simulink library "ROTH"  (R2016b)
settings: Solver=ode45  StartTime=0.0  StopTime=10.0  RelTol=1e-3  EnableMultiTasking=on
undefined symbols (not defined in the file): CAL_EAST, CAL_NORTH, CAL_SOUTH, CAL_WEST, CONST_EndOfLineEnableFlg, ENU_END, ENU_FORWARD, ENU_GTSP, ENU_LEFT_BUSY_RIGHT_BUSY, ENU_LEFT_BUSY_RIGHT_CLEANED, ENU_LEFT_BUSY_RIGHT_EMPTY, ENU_LEFT_CLEANED_RIGHT_BUSY, ENU_LEFT_CLEANED_RIGHT_CLEANED, ENU_LEFT_CLEANED_RIGHT_EMPTY, ENU_LEFT_EMPTY_RIGHT_BUSY, ENU_LEFT_EMPTY_RIGHT_CLEANED, ENU_LEFT_EMPTY_RIGHT_EMPTY, ENU_MOVE_TURN_LEFT, ENU_MOVE_TURN_RIGHT, ENU_MOVE_U_TURN, ENU_MOVE_U_TURN_LEFT, ENU_MOVE_U_TURN_RIGHT, ENU_STOP, ENU_ZIGZAG
settings Model: Creator=oelkawok  LastModifiedBy=oelkawok
settings DataIOCC: LimitDataPoints=on
settings OptimizationCC: LifeSpan=inf
settings DebuggingCC: AllowSymbolicDim=off  SFUnexpectedBacktrackingDiag=warning  SFNoUnconditionalDefaultTransitionDiag=warning  SFExecutionAtInitializationDiag=none
settings GRTTargetCC: TargetLangStandard=C89/C90 (ANSI)  GeneratePreprocessorConditionals=Disable all
settings ConfigComp: CovMetricSettings=dw  CovHtmlReporting=on  CovSaveCumulativeToWorkspaceVar=on  CovSaveSingleToWorkspaceVar=on  CovExternalEMLEnable=off

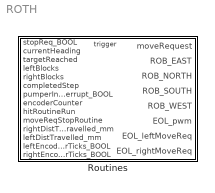
== system ROTH ==
  Routines : Subsystem

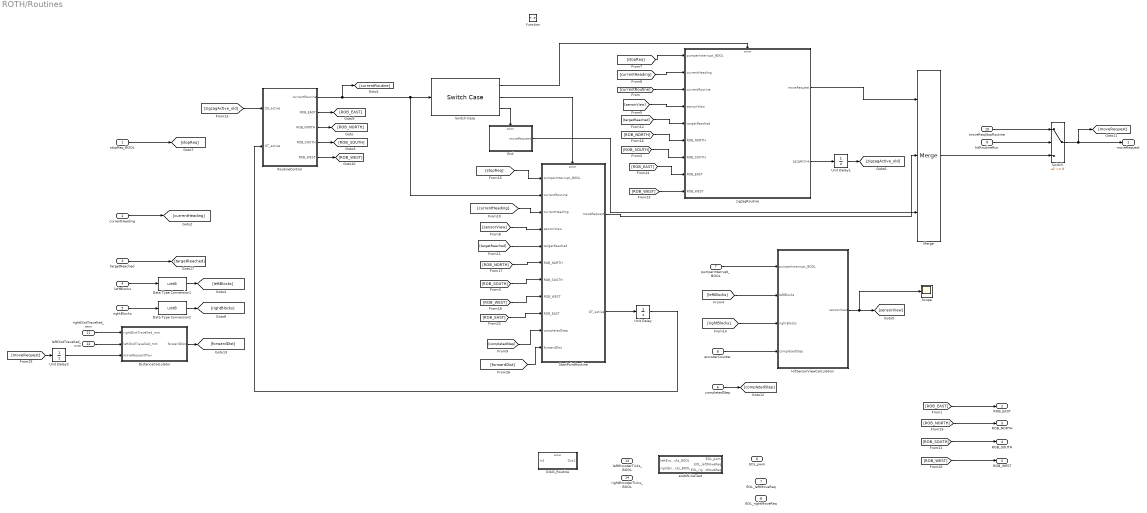
== system ROTH/Routines ==
  stopReq_BOOL : Inport
  currentHeading : Inport  Port=2
  targetReached : Inport  Port=3
  leftBlocks : Inport  Port=4
  rightBlocks : Inport  Port=5
  completedStep : Inport  Port=6
  pumperInterrupt_BOOL : Inport  Port=7
  encoderCounter : Inport  Port=8
  hitRoutineRun : Inport  Port=9
  moveReqStopRoutine : Inport  Port=10
  rightDistTravelled_mm : Inport  Port=11  PortDimensions=1
  leftDistTravelled_mm : Inport  Port=12  PortDimensions=1
  leftEncoderTicks_BOOL : Inport  Port=13  PortDimensions=1
  rightEncoderTicks_BOOL : Inport  Port=14  PortDimensions=1
  function : TriggerPort  TriggerType=function-call  VariantControl=Variant
  DIAG_Routine : Subsystem
  Data Type Conversion1 : DataTypeConversion  OutDataTypeStr=uint8
  Data Type Conversion2 : DataTypeConversion  OutDataTypeStr=uint8
  DistanceCalculator : Subsystem
  End : Subsystem  TreatAsAtomicUnit=on
  HitSensorViewCalculation : Subsystem
  Merge : Merge  Inputs=3  InitialOutput=5
      settings: AttributesFormatString=%<InitialOutput>
  RoutineControl : Subsystem
  Scope : Scope
  StartPointRoutine : Subsystem
  Switch : Switch  Criteria=u2 ~= 0
  Switch Case : SwitchCase  CaseConditions={ENU_ZIGZAG, ENU_GTSP, ENU_END}  ShowDefaultCase=off
      settings: AttributesFormatString=%<CaseConditions>
  Unit Delay : UnitDelay  InitialCondition=true  SampleTime=-1
      settings: AttributesFormatString=%<InitialCondition>
  Unit Delay1 : UnitDelay  InitialCondition=false  SampleTime=-1
      settings: AttributesFormatString=%<InitialCondition>
  Unit Delay2 : UnitDelay  SampleTime=-1
  endofLineTest : Subsystem
  zigzagRoutine : Subsystem
  moveRequest : Outport
  ROB_EAST : Outport  Port=2
  ROB_NORTH : Outport  Port=3
  ROB_SOUTH : Outport  Port=4
  ROB_WEST : Outport  Port=5
  EOL_pwm : Outport  Port=6
  EOL_leftMoveReq : Outport  Port=7
  EOL_rightMoveReq : Outport  Port=8
  wires:
  [forwardDist] -> StartPointRoutine/11(forwardDist)
  DistanceCalculator/1(forwardDist) -> [forwardDist]
  Unit Delay2/1 -> DistanceCalculator/3(moveRequestPrev)
  [moveRequest] -> Unit Delay2/1
  leftDistTravelled_mm/1 -> DistanceCalculator/2(leftDistTravelled_mm)
  rightDistTravelled_mm/1 -> DistanceCalculator/1(rightDistTravelled_mm)
  encoderCounter/1 -> HitSensorViewCalculation/4(completedStep)
  [ROB_WEST] -> zigzagRoutine/9(ROB_WEST)
  [ROB_EAST] -> zigzagRoutine/8(ROB_EAST)
  [completedStep] -> StartPointRoutine/10(completedStep)
  End/1(moveRequest) -> Merge/3
  Switch Case/3 -> End/Action
  [ROB_EAST] -> StartPointRoutine/9(ROB_EAST)
  [ROB_WEST] -> ROB_WEST/1
  [ROB_SOUTH] -> ROB_SOUTH/1
  [ROB_NORTH] -> ROB_NORTH/1
  [ROB_EAST] -> ROB_EAST/1
  [ROB_WEST] -> StartPointRoutine/8(ROB_WEST)
  [ROB_NORTH] -> StartPointRoutine/6(ROB_NORTH)
  [ROB_NORTH] -> zigzagRoutine/6(ROB_NORTH)
  [ROB_SOUTH] -> StartPointRoutine/7(ROB_SOUTH)
  [ROB_SOUTH] -> zigzagRoutine/7(ROB_SOUTH)
  RoutineControl/4(ROB_SOUTH) -> [ROB_SOUTH]
  RoutineControl/5(ROB_WEST) -> [ROB_WEST]
  RoutineControl/2(ROB_EAST) -> [ROB_EAST]
  RoutineControl/3(ROB_NORTH) -> [ROB_NORTH]
  stopReq_BOOL/1 -> [stopReq]
  [targetReached] -> zigzagRoutine/5(targetReached)
  [targetReached] -> StartPointRoutine/5(targetReached)
  targetReached/1 -> [targetReached]
  [currentHeading] -> StartPointRoutine/3(currentHeading)
  [sensorView] -> StartPointRoutine/4(sensorView)
  [stopReq] -> StartPointRoutine/1(pumperInterrupt_BOOL)
  zigzagRoutine/2(zgzgActive) -> Unit Delay1/1
  zigzagRoutine/1(moveRequest) -> Merge/1
  StartPointRoutine/1(moveRequest) -> Merge/2
  pumperInterrupt_BOOL/1 -> HitSensorViewCalculation/1(pumperInterrupt_BOOL)
  Switch Case/2 -> StartPointRoutine/Action
  Switch Case/1 -> zigzagRoutine/Action
  RoutineControl/1(currentRoutine) -> [currentRoutine], Switch Case/1, StartPointRoutine/2(currentRoutine)
  [currentHeading] -> zigzagRoutine/2(currentHeading)
  [stopReq] -> zigzagRoutine/1(pumperInterrupt_BOOL)
  [sensorView] -> zigzagRoutine/4(sensorView)
  HitSensorViewCalculation/1(sensorView) -> Scope/1, [sensorView]
  StartPointRoutine/2(GT_active) -> Unit Delay/1
  Unit Delay/1 -> RoutineControl/2(GT_active)
  currentHeading/1 -> [currentHeading]
  [currentRoutine] -> zigzagRoutine/3(currentRoutine)
  Unit Delay1/1 -> [zigzagActive_old]
  [zigzagActive_old] -> RoutineControl/1(ZG_active)
  leftBlocks/1 -> Data Type Conversion1/1
  rightBlocks/1 -> Data Type Conversion2/1
  Data Type Conversion1/1 -> [leftBlocks]
  Data Type Conversion2/1 -> [rightBlocks]
  [rightBlocks] -> HitSensorViewCalculation/3(rightBlocks)
  [leftBlocks] -> HitSensorViewCalculation/2(leftBlocks)
  completedStep/1 -> [completedStep]
  Switch/1 -> moveRequest/1, [moveRequest]
  moveReqStopRoutine/1 -> Switch/1
  hitRoutineRun/1 -> Switch/2
  Merge/1 -> Switch/3

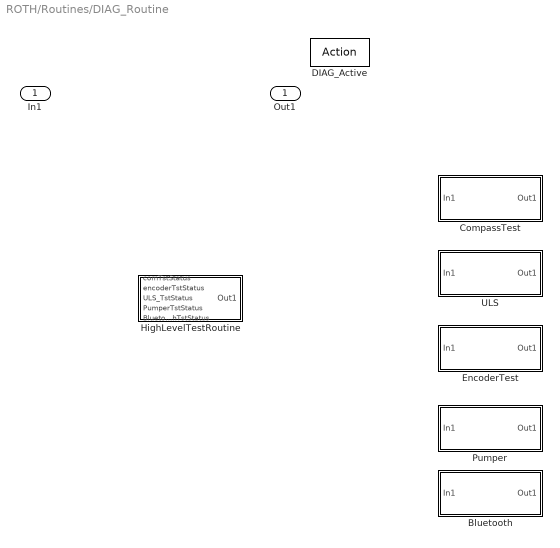
== system ROTH/Routines/DIAG_Routine ==
  In1 : Inport
  DIAG_Active : ActionPort
  Bluetooth : Subsystem
  CompassTest : Subsystem
  EncoderTest : Subsystem
  HighLevelTestRoutine : Subsystem
  Pumper : Subsystem
  ULS : Subsystem
  Out1 : Outport

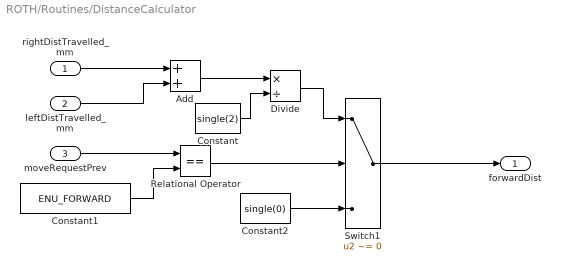
== system ROTH/Routines/DistanceCalculator ==
  rightDistTravelled_mm : Inport  PortDimensions=1
  leftDistTravelled_mm : Inport  Port=2  PortDimensions=1
  moveRequestPrev : Inport  Port=3  PortDimensions=1
  Add : Sum
  Constant : Constant  Value=single(2)
  Constant1 : Constant  Value=ENU_FORWARD
  Constant2 : Constant  Value=single(0)
  Divide : Product  Inputs=*/
  Relational Operator : RelationalOperator  Operator===  OutDataTypeStr=boolean  RndMeth=Simplest
  Switch1 : Switch  Criteria=u2 ~= 0
  forwardDist : Outport
  wires:
  Add/1 -> Divide/1
  moveRequestPrev/1 -> Relational Operator/1
  Constant2/1 -> Switch1/3
  leftDistTravelled_mm/1 -> Add/2
  rightDistTravelled_mm/1 -> Add/1
  Constant1/1 -> Relational Operator/2
  Switch1/1 -> forwardDist/1
  Divide/1 -> Switch1/1
  Relational Operator/1 -> Switch1/2
  Constant/1 -> Divide/2

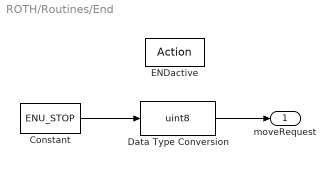
== system ROTH/Routines/End ==
  ENDactive : ActionPort
  Constant : Constant  Value=ENU_STOP
  Data Type Conversion : DataTypeConversion  OutDataTypeStr=uint8
  moveRequest : Outport
  wires:
  Data Type Conversion/1 -> moveRequest/1
  Constant/1 -> Data Type Conversion/1

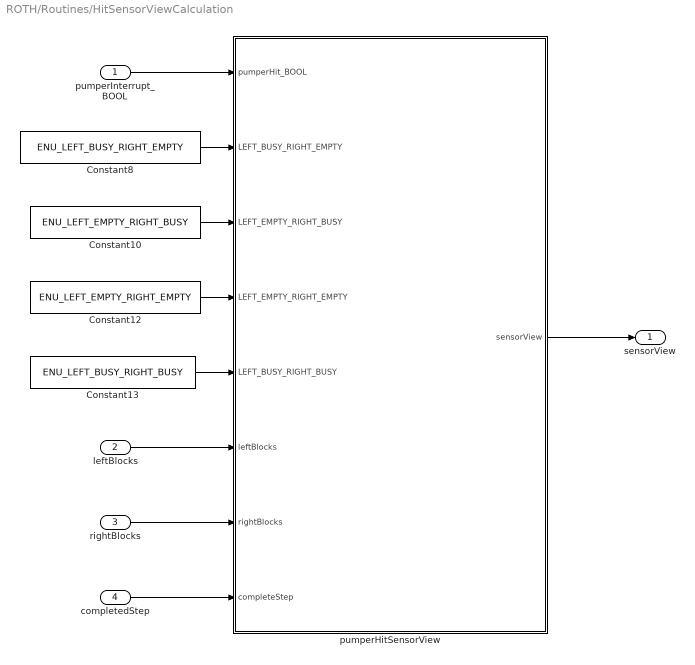
== system ROTH/Routines/HitSensorViewCalculation ==
  pumperInterrupt_BOOL : Inport
  leftBlocks : Inport  Port=2
  rightBlocks : Inport  Port=3
  completedStep : Inport  Port=4
  Constant10 : Constant  Value=ENU_LEFT_EMPTY_RIGHT_BUSY
  Constant12 : Constant  Value=ENU_LEFT_EMPTY_RIGHT_EMPTY
  Constant13 : Constant  Value=ENU_LEFT_BUSY_RIGHT_BUSY
  Constant8 : Constant  Value=ENU_LEFT_BUSY_RIGHT_EMPTY
  pumperHitSensorView : Stateflow chart  TreatAsAtomicUnit=on
  sensorView : Outport
  wires:
  pumperInterrupt_BOOL/1 -> pumperHitSensorView/1(pumperHit_BOOL)
  Constant8/1 -> pumperHitSensorView/2(LEFT_BUSY_RIGHT_EMPTY)
  Constant10/1 -> pumperHitSensorView/3(LEFT_EMPTY_RIGHT_BUSY)
  Constant12/1 -> pumperHitSensorView/4(LEFT_EMPTY_RIGHT_EMPTY)
  Constant13/1 -> pumperHitSensorView/5(LEFT_BUSY_RIGHT_BUSY)
  pumperHitSensorView/1(sensorView) -> sensorView/1
  leftBlocks/1 -> pumperHitSensorView/6(leftBlocks)
  rightBlocks/1 -> pumperHitSensorView/7(rightBlocks)
  completedStep/1 -> pumperHitSensorView/8(completeStep)

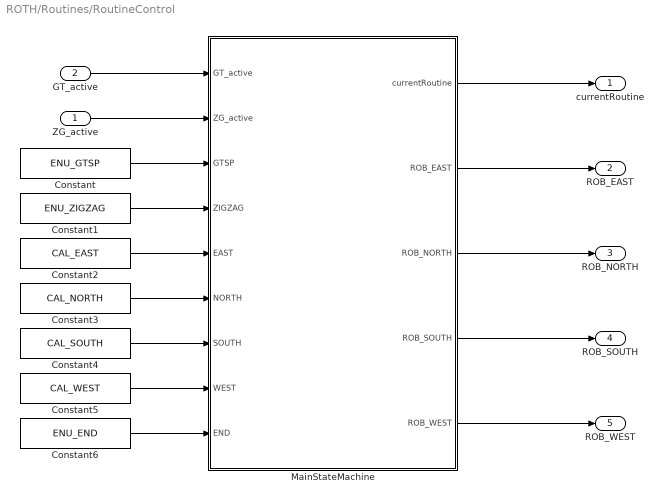
== system ROTH/Routines/RoutineControl ==
  ZG_active : Inport
  GT_active : Inport  Port=2
  Constant : Constant  Value=ENU_GTSP
  Constant1 : Constant  Value=ENU_ZIGZAG
  Constant2 : Constant  Value=CAL_EAST
  Constant3 : Constant  Value=CAL_NORTH
  Constant4 : Constant  Value=CAL_SOUTH
  Constant5 : Constant  Value=CAL_WEST
  Constant6 : Constant  Value=ENU_END
  MainStateMachine : Stateflow chart  TreatAsAtomicUnit=on
  currentRoutine : Outport
  ROB_EAST : Outport  Port=2
  ROB_NORTH : Outport  Port=3
  ROB_SOUTH : Outport  Port=4
  ROB_WEST : Outport  Port=5
  wires:
  Constant6/1 -> MainStateMachine/9(END)
  MainStateMachine/5(ROB_WEST) -> ROB_WEST/1
  MainStateMachine/4(ROB_SOUTH) -> ROB_SOUTH/1
  MainStateMachine/3(ROB_NORTH) -> ROB_NORTH/1
  MainStateMachine/2(ROB_EAST) -> ROB_EAST/1
  Constant4/1 -> MainStateMachine/7(SOUTH)
  Constant3/1 -> MainStateMachine/6(NORTH)
  Constant5/1 -> MainStateMachine/8(WEST)
  Constant2/1 -> MainStateMachine/5(EAST)
  ZG_active/1 -> MainStateMachine/2(ZG_active)
  GT_active/1 -> MainStateMachine/1(GT_active)
  MainStateMachine/1(currentRoutine) -> currentRoutine/1
  Constant/1 -> MainStateMachine/3(GTSP)
  Constant1/1 -> MainStateMachine/4(ZIGZAG)

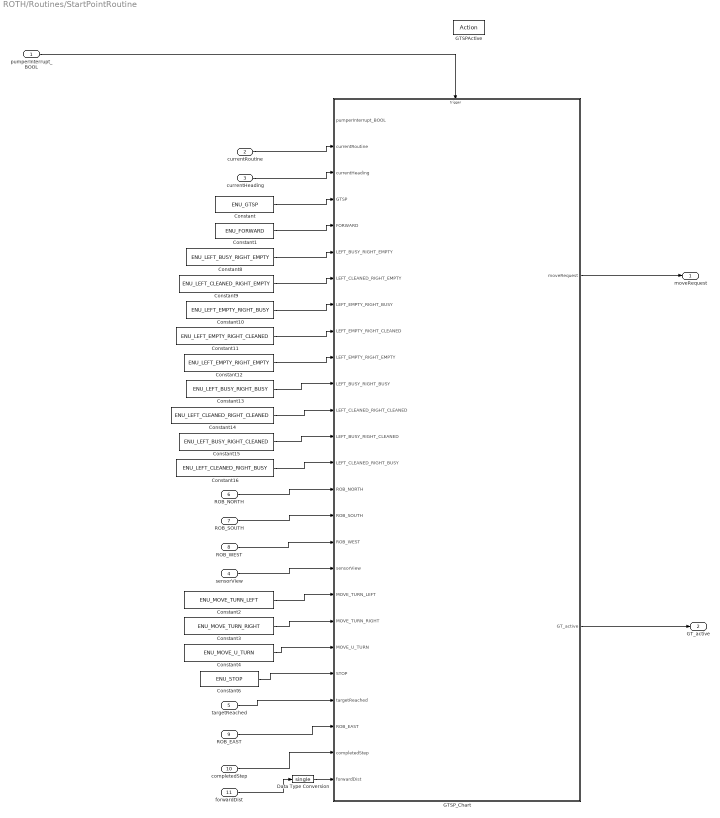
== system ROTH/Routines/StartPointRoutine ==
  pumperInterrupt_BOOL : Inport
  currentRoutine : Inport  Port=2
  currentHeading : Inport  Port=3
  sensorView : Inport  Port=4
  targetReached : Inport  Port=5
  ROB_NORTH : Inport  Port=6
  ROB_SOUTH : Inport  Port=7
  ROB_WEST : Inport  Port=8
  ROB_EAST : Inport  Port=9
  completedStep : Inport  Port=10
  forwardDist : Inport  Port=11
  GTSPActive : ActionPort
  Constant : Constant  Value=ENU_GTSP
  Constant1 : Constant  Value=ENU_FORWARD
  Constant10 : Constant  Value=ENU_LEFT_EMPTY_RIGHT_BUSY
  Constant11 : Constant  Value=ENU_LEFT_EMPTY_RIGHT_CLEANED
  Constant12 : Constant  Value=ENU_LEFT_EMPTY_RIGHT_EMPTY
  Constant13 : Constant  Value=ENU_LEFT_BUSY_RIGHT_BUSY
  Constant14 : Constant  Value=ENU_LEFT_CLEANED_RIGHT_CLEANED
  Constant15 : Constant  Value=ENU_LEFT_BUSY_RIGHT_CLEANED
  Constant16 : Constant  Value=ENU_LEFT_CLEANED_RIGHT_BUSY
  Constant2 : Constant  Value=ENU_MOVE_TURN_LEFT
  Constant3 : Constant  Value=ENU_MOVE_TURN_RIGHT
  Constant4 : Constant  Value=ENU_MOVE_U_TURN
  Constant6 : Constant  Value=ENU_STOP
  Constant8 : Constant  Value=ENU_LEFT_BUSY_RIGHT_EMPTY
  Constant9 : Constant  Value=ENU_LEFT_CLEANED_RIGHT_EMPTY
  Data Type Conversion : DataTypeConversion  OutDataTypeStr=single
  GTSP_Chart : Stateflow chart  TreatAsAtomicUnit=on
  moveRequest : Outport
  GT_active : Outport  Port=2
  wires:
  Data Type Conversion/1 -> GTSP_Chart/26(forwardDist)
  forwardDist/1 -> Data Type Conversion/1
  completedStep/1 -> GTSP_Chart/25(completedStep)
  pumperInterrupt_BOOL/1 -> GTSP_Chart/Trigger
  GTSP_Chart/1(moveRequest) -> moveRequest/1
  ROB_EAST/1 -> GTSP_Chart/24(ROB_EAST)
  targetReached/1 -> GTSP_Chart/23(targetReached)
  currentHeading/1 -> GTSP_Chart/3(currentHeading)
  currentRoutine/1 -> GTSP_Chart/2(currentRoutine)
  Constant/1 -> GTSP_Chart/4(GTSP)
  Constant1/1 -> GTSP_Chart/5(FORWARD)
  Constant8/1 -> GTSP_Chart/6(LEFT_BUSY_RIGHT_EMPTY)
  Constant9/1 -> GTSP_Chart/7(LEFT_CLEANED_RIGHT_EMPTY)
  Constant10/1 -> GTSP_Chart/8(LEFT_EMPTY_RIGHT_BUSY)
  Constant11/1 -> GTSP_Chart/9(LEFT_EMPTY_RIGHT_CLEANED)
  Constant12/1 -> GTSP_Chart/10(LEFT_EMPTY_RIGHT_EMPTY)
  Constant13/1 -> GTSP_Chart/11(LEFT_BUSY_RIGHT_BUSY)
  Constant14/1 -> GTSP_Chart/12(LEFT_CLEANED_RIGHT_CLEANED)
  Constant15/1 -> GTSP_Chart/13(LEFT_BUSY_RIGHT_CLEANED)
  Constant16/1 -> GTSP_Chart/14(LEFT_CLEANED_RIGHT_BUSY)
  ROB_WEST/1 -> GTSP_Chart/17(ROB_WEST)
  ROB_SOUTH/1 -> GTSP_Chart/16(ROB_SOUTH)
  ROB_NORTH/1 -> GTSP_Chart/15(ROB_NORTH)
  sensorView/1 -> GTSP_Chart/18(sensorView)
  Constant4/1 -> GTSP_Chart/21(MOVE_U_TURN)
  Constant3/1 -> GTSP_Chart/20(MOVE_TURN_RIGHT)
  Constant2/1 -> GTSP_Chart/19(MOVE_TURN_LEFT)
  GTSP_Chart/2(GT_active) -> GT_active/1
  Constant6/1 -> GTSP_Chart/22(STOP)

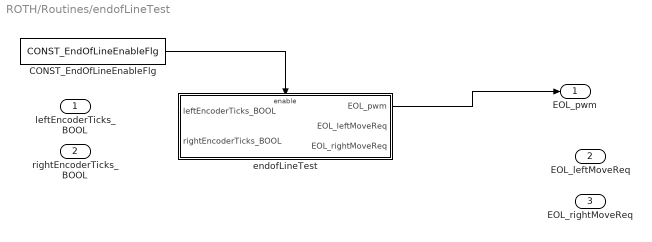
== system ROTH/Routines/endofLineTest ==
  leftEncoderTicks_BOOL : Inport  PortDimensions=1
  rightEncoderTicks_BOOL : Inport  Port=2  PortDimensions=1
  CONST_EndOfLineEnableFlg : Constant  Value=CONST_EndOfLineEnableFlg
  endofLineTest : Subsystem
  EOL_pwm : Outport
  EOL_leftMoveReq : Outport  Port=2
  EOL_rightMoveReq : Outport  Port=3
  wires:
  endofLineTest/1(EOL_pwm) -> EOL_pwm/1
  CONST_EndOfLineEnableFlg/1 -> endofLineTest/Enable

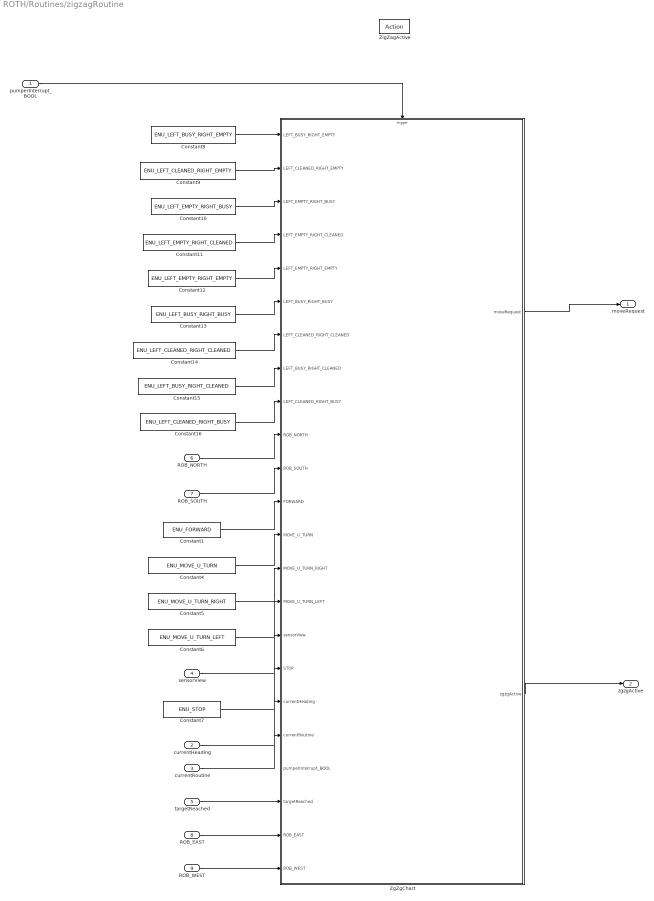
== system ROTH/Routines/zigzagRoutine ==
  pumperInterrupt_BOOL : Inport
  currentHeading : Inport  Port=2
  currentRoutine : Inport  Port=3
  sensorView : Inport  Port=4
  targetReached : Inport  Port=5
  ROB_NORTH : Inport  Port=6
  ROB_SOUTH : Inport  Port=7
  ROB_EAST : Inport  Port=8
  ROB_WEST : Inport  Port=9
  ZigZagActive : ActionPort
  Constant1 : Constant  Value=ENU_FORWARD
  Constant10 : Constant  Value=ENU_LEFT_EMPTY_RIGHT_BUSY
  Constant11 : Constant  Value=ENU_LEFT_EMPTY_RIGHT_CLEANED
  Constant12 : Constant  Value=ENU_LEFT_EMPTY_RIGHT_EMPTY
  Constant13 : Constant  Value=ENU_LEFT_BUSY_RIGHT_BUSY
  Constant14 : Constant  Value=ENU_LEFT_CLEANED_RIGHT_CLEANED
  Constant15 : Constant  Value=ENU_LEFT_BUSY_RIGHT_CLEANED
  Constant16 : Constant  Value=ENU_LEFT_CLEANED_RIGHT_BUSY
  Constant4 : Constant  Value=ENU_MOVE_U_TURN
  Constant5 : Constant  Value=ENU_MOVE_U_TURN_RIGHT
  Constant6 : Constant  Value=ENU_MOVE_U_TURN_LEFT
  Constant7 : Constant  Value=ENU_STOP
  Constant8 : Constant  Value=ENU_LEFT_BUSY_RIGHT_EMPTY
  Constant9 : Constant  Value=ENU_LEFT_CLEANED_RIGHT_EMPTY
  ZgZgChart : Stateflow chart  TreatAsAtomicUnit=on
  moveRequest : Outport
  zgzgActive : Outport  Port=2  InitialOutput=true
  wires:
  ROB_EAST/1 -> ZgZgChart/22(ROB_EAST)
  ROB_WEST/1 -> ZgZgChart/23(ROB_WEST)
  pumperInterrupt_BOOL/1 -> ZgZgChart/Trigger
  ZgZgChart/1(moveRequest) -> moveRequest/1
  targetReached/1 -> ZgZgChart/21(targetReached)
  ZgZgChart/2(zgzgActive) -> zgzgActive/1
  Constant7/1 -> ZgZgChart/17(STOP)
  currentHeading/1 -> ZgZgChart/18(currentHeading)
  currentRoutine/1 -> ZgZgChart/19(currentRoutine)
  sensorView/1 -> ZgZgChart/16(sensorView)
  Constant5/1 -> ZgZgChart/14(MOVE_U_TURN_RIGHT)
  Constant6/1 -> ZgZgChart/15(MOVE_U_TURN_LEFT)
  Constant4/1 -> ZgZgChart/13(MOVE_U_TURN)
  Constant1/1 -> ZgZgChart/12(FORWARD)
  Constant16/1 -> ZgZgChart/9(LEFT_CLEANED_RIGHT_BUSY)
  Constant10/1 -> ZgZgChart/3(LEFT_EMPTY_RIGHT_BUSY)
  Constant12/1 -> ZgZgChart/5(LEFT_EMPTY_RIGHT_EMPTY)
  Constant11/1 -> ZgZgChart/4(LEFT_EMPTY_RIGHT_CLEANED)
  Constant14/1 -> ZgZgChart/7(LEFT_CLEANED_RIGHT_CLEANED)
  ROB_SOUTH/1 -> ZgZgChart/11(ROB_SOUTH)
  ROB_NORTH/1 -> ZgZgChart/10(ROB_NORTH)
  Constant15/1 -> ZgZgChart/8(LEFT_BUSY_RIGHT_CLEANED)
  Constant13/1 -> ZgZgChart/6(LEFT_BUSY_RIGHT_BUSY)
  Constant9/1 -> ZgZgChart/2(LEFT_CLEANED_RIGHT_EMPTY)
  Constant8/1 -> ZgZgChart/1(LEFT_BUSY_RIGHT_EMPTY)

== system ROTH/Routines/DIAG_Routine/Bluetooth ==
  In1 : Inport
  Out1 : Outport
  wires:
  In1/1 -> Out1/1

== system ROTH/Routines/DIAG_Routine/CompassTest ==
  In1 : Inport
  Out1 : Outport
  wires:
  In1/1 -> Out1/1

== system ROTH/Routines/DIAG_Routine/EncoderTest ==
  In1 : Inport
  LeftEncoderTest : Subsystem
  RightEncoderTest : Subsystem
  Out1 : Outport
  wires:
  In1/1 -> Out1/1

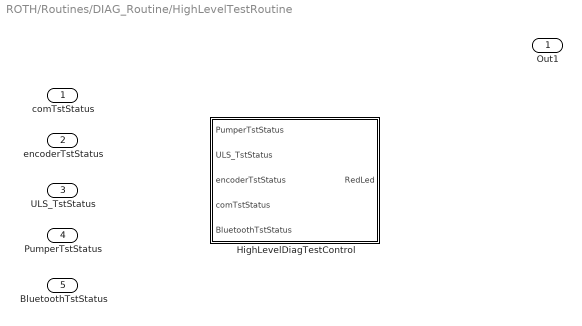
== system ROTH/Routines/DIAG_Routine/HighLevelTestRoutine ==
  comTstStatus : Inport
  encoderTstStatus : Inport  Port=2
  ULS_TstStatus : Inport  Port=3
  PumperTstStatus : Inport  Port=4
  BluetoothTstStatus : Inport  Port=5
  HighLevelDiagTestControl : Stateflow chart  TreatAsAtomicUnit=on
  Out1 : Outport

== system ROTH/Routines/DIAG_Routine/Pumper ==
  In1 : Inport
  Out1 : Outport
  wires:
  In1/1 -> Out1/1

== system ROTH/Routines/DIAG_Routine/ULS ==
  In1 : Inport
  ULSL : Subsystem
  ULSR : Subsystem
  Out1 : Outport
  wires:
  In1/1 -> Out1/1

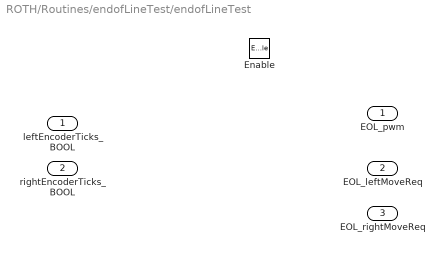
== system ROTH/Routines/endofLineTest/endofLineTest ==
  leftEncoderTicks_BOOL : Inport  PortDimensions=1
  rightEncoderTicks_BOOL : Inport  Port=2  PortDimensions=1
  Enable : EnablePort
  EOL_pwm : Outport
  EOL_leftMoveReq : Outport  Port=2
  EOL_rightMoveReq : Outport  Port=3

== system ROTH/Routines/DIAG_Routine/EncoderTest/LeftEncoderTest ==
  In1 : Inport
  Out1 : Outport
  wires:
  In1/1 -> Out1/1

== system ROTH/Routines/DIAG_Routine/EncoderTest/RightEncoderTest ==
  In1 : Inport
  Out1 : Outport
  wires:
  In1/1 -> Out1/1

== system ROTH/Routines/DIAG_Routine/ULS/ULSL ==
  In1 : Inport
  Out1 : Outport
  wires:
  In1/1 -> Out1/1

== system ROTH/Routines/DIAG_Routine/ULS/ULSR ==
  In1 : Inport
  Out1 : Outport
  wires:
  In1/1 -> Out1/1

== stateflow chart ROTH/Routines/HitSensorViewCalculation/pumperHitSensorView ==
  (default) -> (junction 68) : {
      | //sensorView = 0;
      | }
  (junction 68) -> (junction 69) [order 1] : [pumperHit_BOOL || hasChanged(completeStep)]
  (junction 69) -> (junction 71)
  (junction 68) -> (junction 95) [order 2]
  (junction 71) -> (junction 73) [order 1] : [(leftBlocks <= 1) ...
      | && (rightBlocks >= 1)]
  (junction 71) -> (junction 101) [order 2]
  (junction 73) -> (junction 100) : {
      | sensorView = LEFT_BUSY_RIGHT_EMPTY;
      | }
  (junction 100) -> (junction 101)
  (junction 101) -> (junction 76)
  (junction 76) -> (junction 75) [order 1] : [(leftBlocks >= 1)...
      | && (rightBlocks <= 1)]
  (junction 76) -> (junction 102) [order 2]
  (junction 75) -> (junction 103) : {
      | sensorView = LEFT_EMPTY_RIGHT_BUSY;
      | }
  (junction 103) -> (junction 102)
  (junction 102) -> (junction 78)
  (junction 78) -> (junction 77) [order 1] : [(leftBlocks >= 1)...
      | && (rightBlocks >= 1)]
  (junction 78) -> (junction 104) [order 2]
  (junction 77) -> (junction 105) : {
      | sensorView = LEFT_EMPTY_RIGHT_EMPTY;
      | }
  (junction 105) -> (junction 104)
  (junction 104) -> (junction 80)
  (junction 80) -> (junction 79) [order 1] : [(leftBlocks < 1) ...
      | && (rightBlocks < 1)]
  (junction 80) -> (junction 91) [order 2]
  (junction 79) -> (junction 90) : {
      | sensorView = LEFT_BUSY_RIGHT_BUSY;
      | }
  (junction 91) -> (junction 95)
  (junction 90) -> (junction 91)
  (junction 95) -> (junction 98)
  data: pumperHit_BOOL input; sensorView output uint8; LEFT_BUSY_RIGHT_EMPTY input; LEFT_EMPTY_RIGHT_BUSY input; LEFT_EMPTY_RIGHT_EMPTY input; LEFT_BUSY_RIGHT_BUSY input; leftBlocks input; rightBlocks input; completeStep input

== stateflow chart ROTH/Routines/RoutineControl/MainStateMachine ==
  state GTSP
    entry:
    currentRoutine = GTSP;
  state init
    en:
    zgzgCounter = 0;
  state ZIGZAG
    entry:
    currentRoutine = ZIGZAG;
    zgzgCounter++;
  state End
    en:
    currentRoutine = END;
  (default) -> init
  GTSP -> ZIGZAG : [(GT_active == false) && after(5,tick)]
  init -> GTSP : /ROB_NORTH = NORTH;
      | ROB_SOUTH = SOUTH;
      | ROB_WEST = WEST;
      | ROB_EAST = EAST;
  ZIGZAG -> GTSP [order 2] : [(ZG_active == false)...
      | && after(5, tick)]
      | /ROB_NORTH = WEST;
      | ROB_SOUTH = EAST;
      | ROB_WEST = SOUTH;
      | ROB_EAST = NORTH;
  ZIGZAG -> End [order 1] : [(ZG_active == false)...
      | && (zgzgCounter >= 2)...
      | && after(5 ,tick)]
  data: currentRoutine output uint8; GT_active input; ZG_active input; GTSP input; ZIGZAG input; zgzgCounter local uint8; ROB_EAST output uint16; ROB_NORTH output uint16; ROB_SOUTH output uint16; ROB_WEST output uint16; EAST input; NORTH input; SOUTH input; WEST input; END input

== stateflow chart ROTH/Routines/StartPointRoutine/GTSP_Chart ==
  state Idle
    entry:
    counter = 0;
    moveRequest = STOP;
    step1Flag = false;
    GT_active = true;
    du:
    counter++;
  state GTSP_Active
    state Forward
      entry:
      moveRequest = FORWARD;
    state TurnLeft
      entry:
      moveRequest = MOVE_TURN_LEFT;
    state preFinishLeftBlockedN
      entry:
      moveRequest = MOVE_U_TURN;
    state preFinishLeftBlockedW
      entry:
      moveRequest = MOVE_TURN_RIGHT;
    state preFinishNormal
      entry:
      moveRequest = MOVE_TURN_LEFT;
    state preFinishBlockedW
    state preFinishBlockedN
      entry:
      moveRequest = MOVE_U_TURN;
    state finishedGTSP
      entry:
      step1Flag = true;
      moveRequest = STOP;
    TurnLeft -> Forward : [(currentHeading == ROB_WEST)...
        | && (targetReached == true)]
    (default) -> Forward
    Forward -> (junction 14) : stopEvent
    (junction 14) -> (junction 17) [order 1] : [(sensorView == LEFT_EMPTY_RIGHT_EMPTY)...
        | || (sensorView == LEFT_EMPTY_RIGHT_CLEANED)...
        | || (sensorView == LEFT_EMPTY_RIGHT_BUSY)]
    (junction 14) -> (junction 22) [order 2] : [(sensorView == LEFT_CLEANED_RIGHT_EMPTY)...
        | || (sensorView == LEFT_BUSY_RIGHT_EMPTY)]
    (junction 14) -> (junction 29) [order 3] : [(sensorView == LEFT_BUSY_RIGHT_BUSY)...
        | || (sensorView == LEFT_BUSY_RIGHT_CLEANED)...
        | || (sensorView == LEFT_CLEANED_RIGHT_BUSY)...
        | || (sensorView == LEFT_CLEANED_RIGHT_CLEANED)]
    (junction 17) -> TurnLeft [order 1] : [currentHeading == ROB_NORTH]
    (junction 17) -> preFinishNormal [order 2] : [currentHeading == ROB_WEST]
    (junction 22) -> preFinishLeftBlockedW [order 2] : [currentHeading == ROB_WEST]
    (junction 22) -> preFinishLeftBlockedN [order 1] : [currentHeading == ROB_NORTH]
    (junction 29) -> preFinishBlockedW [order 1] : [currentHeading == ROB_WEST]
    (junction 29) -> preFinishBlockedN [order 2] : [currentHeading == ROB_NORTH]
    preFinishLeftBlockedW -> finishedGTSP : [(currentHeading == ROB_NORTH)...
        | && (targetReached == true)]
    preFinishNormal -> finishedGTSP : [(currentHeading == ROB_SOUTH)...
        | && (targetReached == true)]
    preFinishBlockedN -> finishedGTSP : [(currentHeading == ROB_NORTH)...
        | && (targetReached == true)]
    preFinishBlockedW -> finishedGTSP
  state faceWest
    state turingRight
      entry:
      moveRequest = MOVE_U_TURN;
    state Start
      en:
      initHeading = false;
    state turningLeft
      entry:
      moveRequest = MOVE_TURN_RIGHT;
    state finishInit
      en:
      initHeading = true;
    state uturn
      entry:
      moveRequest = MOVE_TURN_LEFT;
    Start -> turingRight [order 1] : [currentHeading == ROB_SOUTH]
    turingRight -> (junction 135)
    (default) -> Start
    Start -> turningLeft [order 2] : [currentHeading == ROB_WEST]
    Start -> uturn [order 3] : [currentHeading == ROB_EAST]
    turningLeft -> (junction 135)
    (junction 135) -> finishInit : [currentHeading == ROB_NORTH]
    Start -> finishInit [order 4] : [currentHeading == ROB_NORTH]
    uturn -> (junction 135)
  state MostSouthLeft
    state start
    state facingNorth
      state GTSPsearch
        en:
        round = 0;
        state start
          en:
          moveRequest = FORWARD;
          round++;
        state furtherDown
          en:
          moveRequest = MOVE_TURN_LEFT;
        state countingGap
          entry:
          gapCounter = 0;
          du:
          gapCounter++;
        state emptyOnRight
          en:
          moveRequest = MOVE_TURN_RIGHT;
        state facingWest
          en:
          moveRequest = FORWARD;
        (default) -> MostSouthLeft.facingNorth.GTSPsearch.start
        MostSouthLeft.facingNorth.GTSPsearch.start -> MostSouthLeft.facingNorth.GTSPsearch.countingGap [order 2] : [sensorView == LEFT_BUSY_RIGHT_EMPTY...
            | || sensorView == LEFT_EMPTY_RIGHT_EMPTY]
        MostSouthLeft.facingNorth.GTSPsearch.furtherDown -> MostSouthLeft.facingNorth.GTSPsearch.start : [(currentHeading == ROB_SOUTH)...
            | && (targetReached)]
        (junction 123) -> MostSouthLeft.facingNorth.GTSPsearch.furtherDown [order 2] : [(sensorView == LEFT_EMPTY_RIGHT_BUSY)...
            | || (sensorView == LEFT_EMPTY_RIGHT_EMPTY)]
        MostSouthLeft.facingNorth.GTSPsearch.countingGap -> MostSouthLeft.facingNorth.GTSPsearch.emptyOnRight : [(sensorView == LEFT_BUSY_RIGHT_EMPTY...
            | || sensorView == LEFT_EMPTY_RIGHT_EMPTY) ...
            | && (gapCounter >= 100)]
        MostSouthLeft.facingNorth.GTSPsearch.facingWest -> (junction 123) : [pumperInterrupt_BOOL]
            | /moveRequest = STOP;
        MostSouthLeft.facingNorth.GTSPsearch.emptyOnRight -> MostSouthLeft.facingNorth.GTSPsearch.facingWest : [(currentHeading == ROB_WEST)...
            | && (targetReached)]
      state End
        en:
        activeFlag = false;
      (default) -> MostSouthLeft.facingNorth.GTSPsearch
      MostSouthLeft.facingNorth.GTSPsearch -> MostSouthLeft.facingNorth.End : [(currentHeading == ROB_SOUTH)...
          | && (targetReached)...
          | && (pumperInterrupt_BOOL)...
          | && (round > 1)]
          | /moveRequest = STOP;
      MostSouthLeft.facingNorth.GTSPsearch.start -> MostSouthLeft.facingNorth.End [order 1] : [pumperInterrupt_BOOL]
          | /moveRequest = STOP;
      (junction 123) -> MostSouthLeft.facingNorth.End [order 1] : [(sensorView == LEFT_BUSY_RIGHT_BUSY)...
          | || (sensorView == LEFT_BUSY_RIGHT_EMPTY)]
    state finish
      en:
      GT_active = false;
    state facingSouth
      state GTSPsearch
        en:
        round = 0;
        state start
          en:
          moveRequest = FORWARD;
          round++;
        state furtherDown
          en:
          moveRequest = MOVE_TURN_LEFT;
        state intermediate
          en:
          tempDist = forwardDist;
        state countingGap
          entry:
          gapCounter = 0;
          du:
          gapCounter++;
        state emptyOnRight
          en:
          moveRequest = MOVE_TURN_RIGHT;
        state facingWest
          en:
          moveRequest = FORWARD;
        (default) -> MostSouthLeft.facingSouth.GTSPsearch.start
        MostSouthLeft.facingSouth.GTSPsearch.start -> intermediate [order 2] : [(sensorView == LEFT_BUSY_RIGHT_EMPTY...
            | || sensorView == LEFT_EMPTY_RIGHT_EMPTY)]
            | /northCounter = 0;
        intermediate -> MostSouthLeft.facingSouth.GTSPsearch.start [order 1] : [(sensorView != LEFT_BUSY_RIGHT_EMPTY...
            | && sensorView != LEFT_EMPTY_RIGHT_EMPTY)]
        MostSouthLeft.facingSouth.GTSPsearch.start -> (junction 162) [order 1] : stopEvent
        MostSouthLeft.facingSouth.GTSPsearch.furtherDown -> MostSouthLeft.facingSouth.GTSPsearch.start : [(currentHeading == ROB_SOUTH)...
            | && (targetReached)]
        (junction 88) -> MostSouthLeft.facingSouth.GTSPsearch.furtherDown [order 2] : [(sensorView == LEFT_EMPTY_RIGHT_BUSY)...
            | || (sensorView == LEFT_EMPTY_RIGHT_EMPTY)]
        intermediate -> MostSouthLeft.facingSouth.GTSPsearch.emptyOnRight [order 2] : [(forwardDist - tempDist) > CAL_ROBO_LENG_mm]//* 0.75)]
        (junction 162) -> MostSouthLeft.facingSouth.GTSPsearch.emptyOnRight : [(sensorView == LEFT_BUSY_RIGHT_EMPTY...
            | || sensorView == LEFT_EMPTY_RIGHT_EMPTY)]
        MostSouthLeft.facingSouth.GTSPsearch.countingGap -> MostSouthLeft.facingSouth.GTSPsearch.emptyOnRight : [(sensorView == LEFT_BUSY_RIGHT_EMPTY...
            | || sensorView == LEFT_EMPTY_RIGHT_EMPTY) ...
            | && (gapCounter >= CAL_GTSPgapCounter)]
        MostSouthLeft.facingSouth.GTSPsearch.facingWest -> (junction 88) : stopEvent
        MostSouthLeft.facingSouth.GTSPsearch.emptyOnRight -> MostSouthLeft.facingSouth.GTSPsearch.facingWest : [(currentHeading == ROB_WEST)...
            | && (targetReached)]
      state End
        en:
        activeFlag = false;
      (default) -> MostSouthLeft.facingSouth.GTSPsearch
      MostSouthLeft.facingSouth.GTSPsearch -> (junction 154) : stopEvent
      (junction 154) -> MostSouthLeft.facingSouth.End : [(currentHeading == ROB_SOUTH)...
          | && (targetReached)...
          | && (round > 1)] {hitCounter > 3}...
          | /moveRequest = STOP;
      MostSouthLeft.facingSouth.GTSPsearch.start -> MostSouthLeft.facingSouth.End [order 3] : stopEvent
      (junction 88) -> MostSouthLeft.facingSouth.End [order 1] : [(sensorView == LEFT_BUSY_RIGHT_BUSY)...
          | || (sensorView == LEFT_BUSY_RIGHT_EMPTY)]
    (default) -> MostSouthLeft.start
    MostSouthLeft.start -> finish [order 2] : [currentHeading == ROB_NORTH]
    MostSouthLeft.start -> facingSouth [order 1] : [currentHeading == ROB_SOUTH]
    facingNorth -> finish : [activeFlag == false]
    facingSouth -> finish : [activeFlag == false]
  (default) -> Idle
  Idle -> faceWest : [(currentRoutine == GTSP)...
      | && (counter > CAL_GTSPdelayStart)]
  faceWest -> GTSP_Active : [initHeading == true]
  finish -> Idle : [currentRoutine == GTSP]
  GTSP_Active -> Idle [order 1] : [currentRoutine != GTSP]
  GTSP_Active -> MostSouthLeft [order 2] : [step1Flag == true]
      | /activeFlag = true;
  preFinishLeftBlockedN -> (junction 156) : [(currentHeading == ROB_SOUTH)...
      | && (targetReached == true)]
  (junction 156) -> finish
  data: pumperInterrupt_BOOL input; currentRoutine input; currentHeading input; GTSP input; FORWARD input; LEFT_BUSY_RIGHT_EMPTY input; LEFT_CLEANED_RIGHT_EMPTY input; LEFT_EMPTY_RIGHT_BUSY input; LEFT_EMPTY_RIGHT_CLEANED input; LEFT_EMPTY_RIGHT_EMPTY input; LEFT_BUSY_RIGHT_BUSY input; LEFT_CLEANED_RIGHT_CLEANED input; LEFT_BUSY_RIGHT_CLEANED input; LEFT_CLEANED_RIGHT_BUSY input; ROB_NORTH input; ROB_SOUTH input; ROB_WEST input; sensorView input; moveRequest output uint8; MOVE_TURN_LEFT input; MOVE_TURN_RIGHT input; MOVE_U_TURN input; GT_active output boolean =true; STOP input; targetReached input; counter local uint8; gapCounter local uint8; round local uint8; step1Flag local uint8; initHeading local boolean; ROB_EAST input; activeFlag local boolean; CAL_GTSPdelayStart constant uint8 =CAL_GTSPdelayStart; CAL_GTSPgapCounter constant uint8 =CAL_GTSPgapCounter; completedStep input; CAL_SingleStepTicks constant uint8 =CAL_SingleStepTicks; forwardDist input; northCounter local uint8; CAL_ROBO_LENG_mm constant uint16 =uint16(CAL_ROBO_LENG_mm); tempDist local uint16; hitCounter local uint8
  events: refreshEvent input EITHER_EDGE_EVENT; stopEvent input EITHER_EDGE_EVENT

== stateflow chart ROTH/Routines/zigzagRoutine/ZgZgChart ==
  state SwitchLane
  state finishZigZag
    en:
    zgzgActive = false;
    moveRequest = STOP;
  state MovingForward
    en:
    moveRequest = FORWARD;
  state Idle
    en:
    zgzgActive = true;
    finishCounter = 1;
  state faceWest
    state turingRight
      entry:
      moveRequest = MOVE_U_TURN;
    state Start
      en:
      initHeading = false;
    state turningLeft
      entry:
      moveRequest = MOVE_TURN_RIGHT;
    state finishInit
      en:
      initHeading = true;
    state uturn
      entry:
      moveRequest = MOVE_TURN_LEFT;
    Start -> turingRight [order 1] : [currentHeading == ROB_SOUTH]
    turingRight -> (junction 93)
    (default) -> Start
    Start -> turningLeft [order 2] : [currentHeading == ROB_WEST]
    Start -> uturn [order 3] : [currentHeading == ROB_EAST]
    turningLeft -> (junction 93)
    (junction 93) -> finishInit : [currentHeading == ROB_NORTH]
    Start -> finishInit [order 4] : [currentHeading == ROB_NORTH]
    uturn -> (junction 93)
  (junction 34) -> SwitchLane [order 1] : [currentHeading == ROB_NORTH]
      | /moveRequest = MOVE_U_TURN_RIGHT;
      | headingRequest = ROB_SOUTH;
      | finishCounter = 1;
  (junction 34) -> SwitchLane [order 2] : [currentHeading == ROB_SOUTH]
      | /moveRequest = MOVE_U_TURN_LEFT;
      | headingRequest = ROB_NORTH;
      | finishCounter = 1;
  (junction 35) -> SwitchLane [order 1] : [currentHeading == ROB_NORTH]
      | /moveRequest = MOVE_U_TURN_RIGHT;
      | headingRequest = ROB_SOUTH;
      | finishCounter = 1;
  (junction 33) -> (junction 34) [order 1] : [sensorView == LEFT_EMPTY_RIGHT_EMPTY]
  SwitchLane -> finishZigZag [order 1] : [finishCounter > CAL_ZgZgCounterThd]
  (junction 35) -> SwitchLane [order 2] : [currentHeading == ROB_SOUTH]
      | /moveRequest = MOVE_U_TURN;
      | headingRequest = ROB_NORTH;
      | finishCounter++;
  (junction 33) -> (junction 35) [order 2] : [(sensorView == LEFT_CLEANED_RIGHT_EMPTY)...
      | || (sensorView == LEFT_BUSY_RIGHT_EMPTY)]
  MovingForward -> faceWest [order 2] : [currentHeading == ROB_WEST || currentHeading == ROB_EAST]
  (junction 36) -> SwitchLane [order 2] : [currentHeading == ROB_SOUTH]
      | /moveRequest = MOVE_U_TURN_LEFT;
      | headingRequest = ROB_NORTH;
      | finishCounter = 1;
  (default) -> Idle
  finishZigZag -> Idle : [(currentRoutine == ENU_ZIGZAG)]
  MovingForward -> (junction 33) [order 1] : stopEvent
  (junction 36) -> SwitchLane [order 1] : [currentHeading == ROB_NORTH]
      | /moveRequest = MOVE_U_TURN;
      | headingRequest = ROB_SOUTH;
      | finishCounter++;
  faceWest -> MovingForward : [initHeading]
  Idle -> faceWest : [currentRoutine == ENU_ZIGZAG]
  (junction 33) -> (junction 36) [order 4] : [(sensorView == LEFT_EMPTY_RIGHT_CLEANED)...
      | || (sensorView == LEFT_EMPTY_RIGHT_BUSY)]
  (junction 33) -> (junction 37) [order 3] : [(sensorView == LEFT_BUSY_RIGHT_BUSY)]
  (junction 33) -> (junction 37) [order 5] : [(sensorView == LEFT_BUSY_RIGHT_CLEANED)...
      | || (sensorView == LEFT_CLEANED_RIGHT_BUSY)...
      | || (sensorView == LEFT_CLEANED_RIGHT_CLEANED)]
  SwitchLane -> MovingForward [order 2] : [(headingRequest == currentHeading)...
      | && (targetReached == true)]
  (junction 37) -> SwitchLane [order 1] : [currentHeading == ROB_NORTH]
      | /moveRequest = MOVE_U_TURN;
      | headingRequest = ROB_SOUTH;
      | finishCounter++;
  (junction 37) -> SwitchLane [order 2] : [currentHeading == ROB_SOUTH]
      | /moveRequest = MOVE_U_TURN;
      | headingRequest = ROB_NORTH;
      | finishCounter++;
  data: LEFT_BUSY_RIGHT_EMPTY input; LEFT_CLEANED_RIGHT_EMPTY input; LEFT_EMPTY_RIGHT_BUSY input; LEFT_EMPTY_RIGHT_CLEANED input; LEFT_EMPTY_RIGHT_EMPTY input; LEFT_BUSY_RIGHT_BUSY input; LEFT_CLEANED_RIGHT_CLEANED input; LEFT_BUSY_RIGHT_CLEANED input; LEFT_CLEANED_RIGHT_BUSY input; ROB_NORTH input; ROB_SOUTH input; FORWARD input; MOVE_U_TURN input; MOVE_U_TURN_RIGHT input; MOVE_U_TURN_LEFT input; sensorView input; STOP input; moveRequest output uint8; currentHeading input; currentRoutine input; pumperInterrupt_BOOL input; targetReached input; headingRequest local uint16; ENU_ZIGZAG parameter; zgzgActive output boolean =true;; finishCounter local uint8; CAL_ZgZgCounterThd constant uint8 =CAL_ZgZgCounterThd; initHeading local double; MOVE_TURN_LEFT constant uint8 =ENU_MOVE_TURN_LEFT; MOVE_TURN_RIGHT constant uint8 =ENU_MOVE_TURN_RIGHT; ROB_EAST input =CAL_ROB_EAST; ROB_WEST input =CAL_ROB_WEST
  events: refreshEvent input EITHER_EDGE_EVENT; stopEvent input EITHER_EDGE_EVENT

== stateflow chart ROTH/Routines/DIAG_Routine/HighLevelTestRoutine/HighLevelDiagTestControl ==
  state Failed
    en:
    RedLed = true;
  state CompassRoutine
  state EncoderRoutine
  state ULS_Routine
  state PumperRoutine
  state BlueTooth
  (default) -> CompassRoutine
  CompassRoutine -> Failed [order 2] : [comTstStatus == ENU_FAILED]
  CompassRoutine -> EncoderRoutine [order 1] : [comTstStatus == ENU_PASSED]
  EncoderRoutine -> Failed [order 2] : [encoderTstStatus == ENU_FAILED]
  EncoderRoutine -> ULS_Routine [order 1] : [encoderTstStatus == ENU_PASSED]
  ULS_Routine -> Failed [order 2] : [ULS_TstStatus == ENU_FAILED]
  ULS_Routine -> PumperRoutine [order 1] : [ULS_TstStatus == ENU_PASSED]
  PumperRoutine -> Failed [order 2] : [PumperTstStatus == ENU_FAILED]
  PumperRoutine -> BlueTooth [order 1] : [PumperTstStatus == ENU_PASSED]
  BlueTooth -> Failed : [BluetoothTstStatus == ENU_FAILED]
  data: PumperTstStatus input; ULS_TstStatus input; encoderTstStatus input; RedLed output double; ENU_FAILED constant uint8 =ENU_FAILED; comTstStatus input; BluetoothTstStatus input; ENU_PASSED constant uint8 =ENU_PASSED
